simulink model "ColorCoded"  (R2017b)
settings: Solver=VariableStepAuto  StartTime=0.0  StopTime=10.0  RelTol=1e-3
settings Model: Creator=E3I4N1V  LastModifiedBy=E3I4N1V

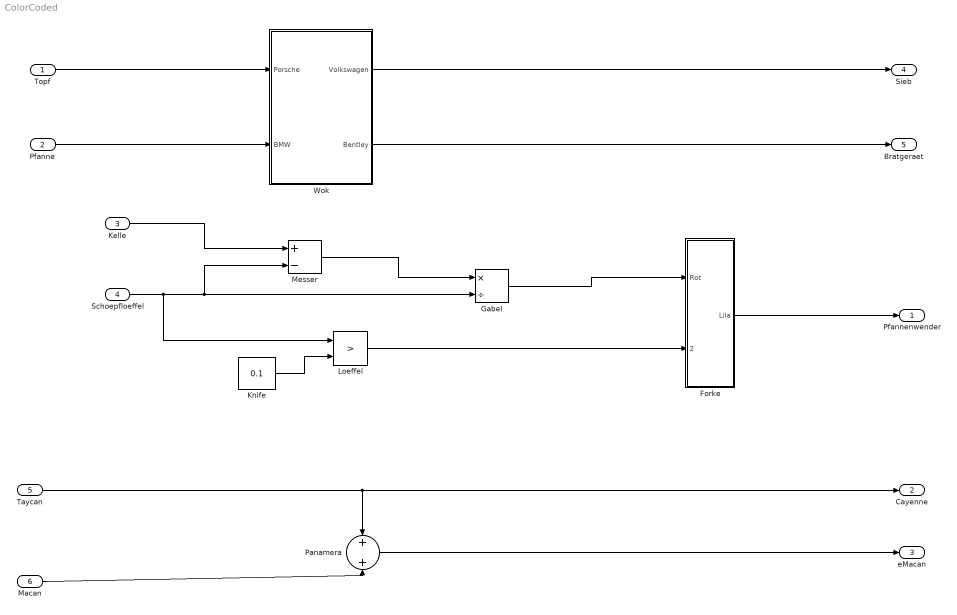
== system ColorCoded ==
  Topf : Inport
  Pfanne : Inport  Port=2
  Kelle : Inport  Port=3
  Schoepfloeffel : Inport  Port=4
  Taycan : Inport  Port=5
  Macan : Inport  Port=6
  Forke : Subsystem
  Gabel : Product  Inputs=*/  RndMeth=Zero
  Knife : Constant  Value=0.1
  Loeffel : RelationalOperator  Operator=>  OutDataTypeStr=boolean  RndMeth=Nearest
  Messer : Sum  Inputs=+-
  Panamera : Sum
  Wok : Subsystem
  Pfannenwender : Outport
  Cayenne : Outport  Port=2
  eMacan : Outport  Port=3
  Sieb : Outport  Port=4
  Bratgeraet : Outport  Port=5
  wires:
  Pfanne/1 -> Wok/2(BMW)
  Topf/1 -> Wok/1(Porsche)
  Kelle/1 -> Messer/1
  Schoepfloeffel/1 -> Loeffel/1, Gabel/2, Messer/2
  Messer/1 -> Gabel/1
  Knife/1 -> Loeffel/2
  Taycan/1 -> Panamera/1, Cayenne/1
  Macan/1 -> Panamera/2
  Panamera/1 -> eMacan/1
  Wok/2(Bentley) -> Bratgeraet/1
  Wok/1(Volkswagen) -> Sieb/1
  Gabel/1 -> Forke/1(Rot)
  Loeffel/1 -> Forke/2(Orange)
  Forke/1(Lila) -> Pfannenwender/1

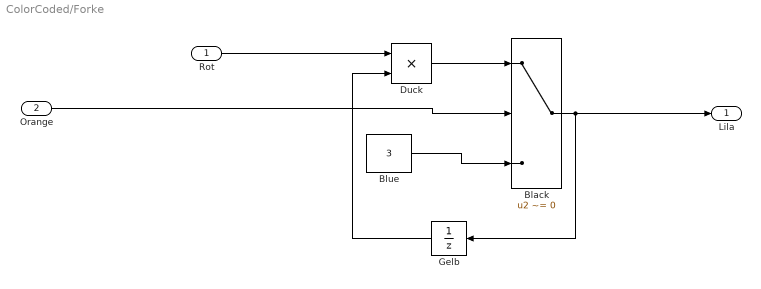
== system ColorCoded/Forke ==
  Rot : Inport
  Orange : Inport  Port=2
  Black : Switch  Criteria=u2 ~= 0
  Blue : Constant  Value=3
  Duck : Product  Inputs=**  RndMeth=Zero
  Gelb : UnitDelay  SampleTime=-1
  Lila : Outport
  wires:
  Rot/1 -> Duck/1
  Black/1 -> Lila/1, Gelb/1
  Duck/1 -> Black/1
  Orange/1 -> Black/2
  Blue/1 -> Black/3
  Gelb/1 -> Duck/2

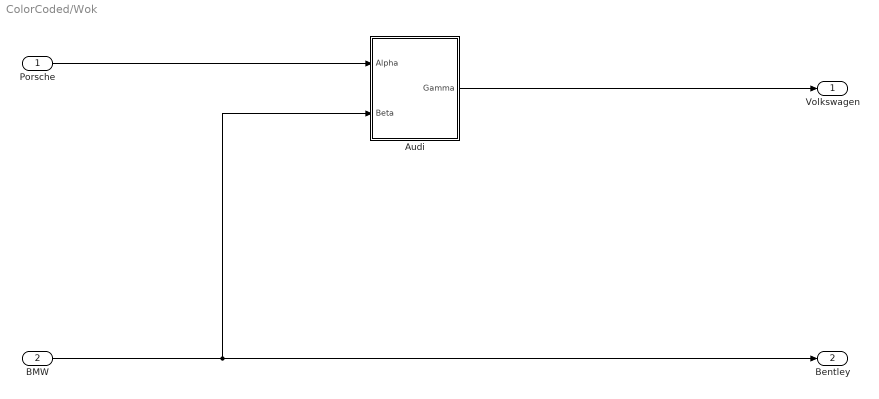
== system ColorCoded/Wok ==
  Porsche : Inport
  BMW : Inport  Port=2
  Audi : Subsystem
  Volkswagen : Outport
  Bentley : Outport  Port=2
  wires:
  BMW/1 -> Audi/2(Beta), Bentley/1
  Porsche/1 -> Audi/1(Alpha)
  Audi/1(Gamma) -> Volkswagen/1

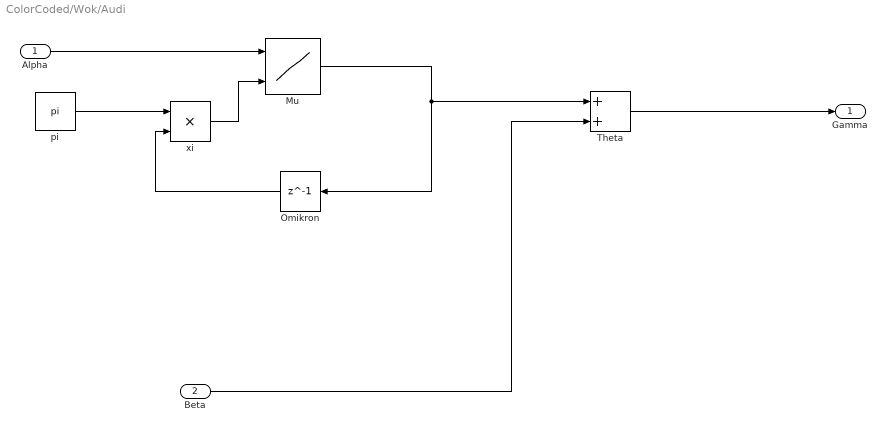
== system ColorCoded/Wok/Audi ==
  Alpha : Inport
  Beta : Inport  Port=2
  Mu : Lookup_n-D  BreakpointsForDimension1=[1:3]  BreakpointsForDimension2=[1:3]  IndexSearchMethod=Linear search  ExtrapMethod=Clip  InternalRulePriority=Speed  RndMeth=Simplest  InputSameDT=on
  Omikron : Delay  DelayLength=1  InitialCondition=0
  Theta : Sum
  pi : Constant  Value=pi
  xi : Product  Inputs=**  RndMeth=Zero
  Gamma : Outport
  wires:
  Alpha/1 -> Mu/1
  Omikron/1 -> xi/2
  Theta/1 -> Gamma/1
  Beta/1 -> Theta/2
  Mu/1 -> Theta/1, Omikron/1
  pi/1 -> xi/1
  xi/1 -> Mu/2
